simulink model "Transformation"  (R2021b)
settings: Solver=VariableStepAuto  StartTime=0.0  StopTime=10.0  RelTol=1e-3
libraries: aerolibutil x3, aerosimlib x1, sharedutil x1, sharedtransform x1
settings Model: Creator=SuturinDA  LastModifiedBy=SuturinDA

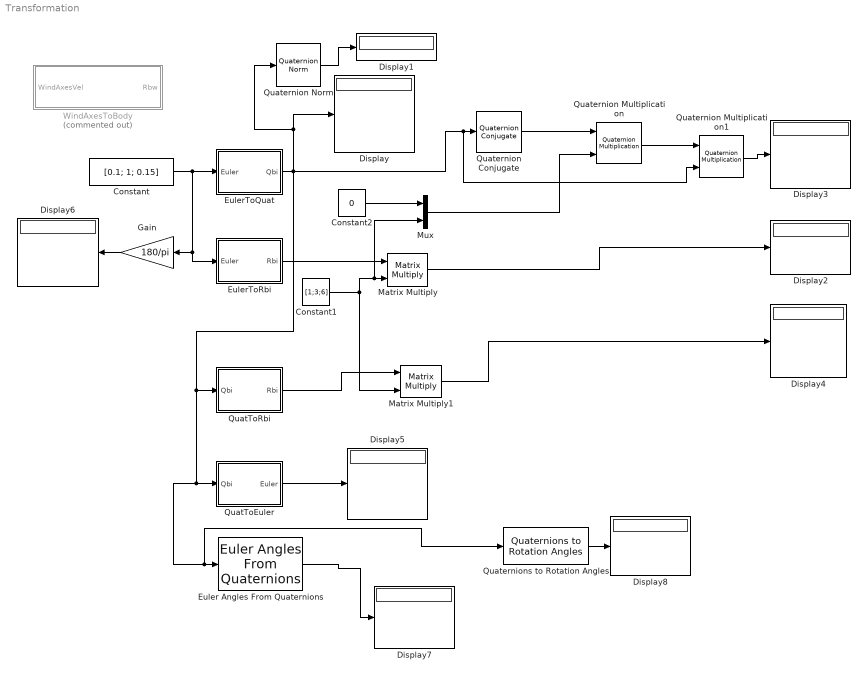
== system Transformation ==
  Constant : Constant  Value=[0.1; 1; 0.15]
  Constant1 : Constant  Value=[1;3;6]
  Constant2 : Constant  Value=0
  Display{,1..8} (9 alike) : Display
  Euler Angles From Quaternions : aerosimlib/Transformations/Euler Angles From Quaternions
  EulerToQuat : MATLAB Function  TreatAsAtomicUnit=on
  EulerToRbi : MATLAB Function  TreatAsAtomicUnit=on
  Gain : Gain  Gain=180/pi
  Matrix Multiply : Product  Multiplication=Matrix(*)
  Matrix Multiply1 : Product  Multiplication=Matrix(*)
  Mux : Mux  Inputs=2
  QuatToEuler : MATLAB Function  TreatAsAtomicUnit=on
  QuatToRbi : MATLAB Function  TreatAsAtomicUnit=on
  Quaternion Conjugate : aerolibutil/Quaternion Conjugate
      settings: SourceProductBaseCode=AE
  Quaternion Multiplication : aerolibutil/Quaternion Multiplication
  Quaternion Multiplication1 : aerolibutil/Quaternion Multiplication
  Quaternion Norm : sharedutil/Quaternion Norm  aMode=aMode
      settings: SourceProductBaseCode=AE,PW,DR,MT,UV,VE
  Quaternions to Rotation Angles : sharedtransform/Quaternions to Rotation Angles  rotationOrder=XYZ  aMode=aMode
      settings: SourceProductBaseCode=AE,PW,DR,MT,UV,VE
  WindAxesToBody : MATLAB Function  Commented=on  TreatAsAtomicUnit=on
  wires:
  Constant/1 -> EulerToRbi/1(Euler), Gain/1, EulerToQuat/1(Euler)
  EulerToQuat/1(Qbi) -> Quaternion Multiplication1/2, Quaternion Conjugate/1, Display/1, Quaternion Norm/1, QuatToEuler/1(Qbi), Quaternions to Rotation Angles/1, Euler Angles From Quaternions/1, QuatToRbi/1(Qbi)
  Quaternion Norm/1 -> Display1/1
  EulerToRbi/1(Rbi) -> Matrix Multiply/1
  Constant1/1 -> Matrix Multiply1/2, Mux/2, Matrix Multiply/2
  Matrix Multiply/1 -> Display2/1
  Constant2/1 -> Mux/1
  Quaternion Conjugate/1 -> Quaternion Multiplication/1
  Mux/1 -> Quaternion Multiplication/2
  Quaternion Multiplication/1 -> Quaternion Multiplication1/1
  Quaternion Multiplication1/1 -> Display3/1
  QuatToRbi/1(Rbi) -> Matrix Multiply1/1
  Matrix Multiply1/1 -> Display4/1
  QuatToEuler/1(Euler) -> Display5/1
  Gain/1 -> Display6/1
  Euler Angles From Quaternions/1 -> Display7/1
  Quaternions to Rotation Angles/1 -> Display8/1

== matlab function Transformation/WindAxesToBody ==
  data: WindAxesVel input; Rbw output
function Rbw = fcn(WindAxesVel)

Va = WindAxesVel(1);
a = WindAxesVel(2);
b = WindAxesVel(3);

Rbs = [[cos(a) 0 -sin(a)];
    [0 1 0];
    [sin(a) 0 cos(a)]];

Rws = [[cos(b) sin(b) 0];
    [-sin(b) cos(b) 0];
    [0 0 1]];

Rbw = Rbs * Rws';
end

== matlab function Transformation/EulerToQuat ==
  data: Euler input; Qbi output
function Qbi = fcn(Euler)

phi = Euler(1);
theta = Euler(2);
psi = Euler(3);

q1 = [cos(psi/2) 0 0 sin(psi/2)];
q2 = [cos(theta/2) 0 sin(theta/2) 0];
q3 = [cos(phi/2) sin(phi/2) 0 0];

Qib = quatmultiply(quatmultiply(q1, q2), q3);

tempQbi = quatconj(Qib);

Qbi = reshape(tempQbi, 4, 1);
end

== matlab function Transformation/QuatToRbi ==
  data: Qbi input; Rbi output
function Rbi = fcn(Qbi)

q0 = Qbi(1);
q1 = Qbi(2);
q2 = Qbi(3);
q3 = Qbi(4);

Rbi = [[(1-2*q2*q2-2*q3*q3) 2*(q1*q2+q3*q0) 2*(q1*q3-q0*q2)];
    [2*(q1*q2-q3*q0) (q0*q0+q2*q2-q1*q1-q3*q3) 2*(q2*q3+q1*q0)];
    [2*(q1*q3+q0*q2) 2*(q2*q3-q1*q0) (q0*q0+q3*q3-q1*q1-q2*q2)]];

== matlab function Transformation/QuatToEuler ==
  data: Qbi input; Euler output
function Euler = fcn(Qbi)

q0 = Qbi(1);
q1 = Qbi(2);
q2 = Qbi(3);
q3 = Qbi(4);

phi = atan2(2*(q0*q1+q2*q3), (q0*q0+q3*q3-q1*q1-q2*q2));
theta = asin(2*(q0*q2-q1*q3));
psi = atan2(2*(q0*q3+q1*q2), (q0*q0+q1*q1-q2*q2-q3*q3));

phi = mod(phi + pi, 2*pi) - pi;
theta = mod(theta + pi, 2*pi) - pi;
psi = mod(psi + pi, 2*pi) - pi;

Euler = [phi; theta; psi];

end

== matlab function Transformation/EulerToRbi ==
  data: Euler input; Rbi output
function Rbi = fcn( Euler)

phi = Euler(1);
theta = Euler(2);
psi = Euler(3);

R1 = [[cos(psi) sin(psi) 0];
    [-sin(psi) cos(psi) 0];
    [0 0 1]];

R2 = [[cos(theta) 0 -sin(theta)];
    [0 1 0];
    [sin(theta) 0 cos(theta)]];

R3 = [[1 0 0];
    [0 cos(phi) sin(phi)];
    [0 -sin(phi) cos(phi)]];

Rib = R3*R2*R1;
Rbi = Rib';
end
